simulink model "Bicycle_Rebuild"  (R2019b)
settings: Solver=VariableStepAuto  StartTime=0.0  StopTime=20  MaxStep=1e-3  RelTol=1e-3
values from neighbouring files (symbols this model uses):
  K = lqr(A,B,Q,R)    [Lqr.m]
undefined symbols (not defined in the file or in its folder): DC_Motor, Dynamics, Theta
settings Model: Creator=user  LastModifiedBy=user

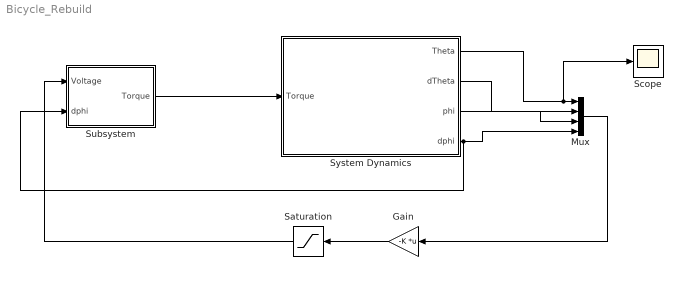
== system Bicycle_Rebuild ==
  Gain : Gain  Gain=-K  Multiplication=Matrix(K*u)
  Mux : Mux
  Saturation : Saturate  UpperLimit=24  LowerLimit=-24
  Scope : Scope
  Subsystem : Subsystem
  System Dynamics : Subsystem
  wires:
  Subsystem/1(Torque) -> System Dynamics/1(Torque)
  System Dynamics/4(dphi) -> Subsystem/2(dphi), Mux/4
  Mux/1 -> Gain/1
  System Dynamics/3(phi) -> Mux/3
  System Dynamics/2(dTheta) -> Mux/2
  System Dynamics/1(Theta) -> Scope/1, Mux/1
  Gain/1 -> Saturation/1
  Saturation/1 -> Subsystem/1(Voltage)

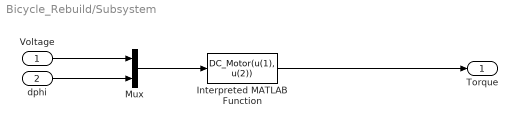
== system Bicycle_Rebuild/Subsystem ==
  Voltage : Inport
  dphi : Inport  Port=2
  Interpreted MATLAB Function : MATLABFcn  MATLABFcn=DC_Motor(u(1), u(2))
  Mux : Mux  Inputs=2
  Torque : Outport
  wires:
  dphi/1 -> Mux/2
  Interpreted MATLAB Function/1 -> Torque/1
  Mux/1 -> Interpreted MATLAB Function/1
  Voltage/1 -> Mux/1

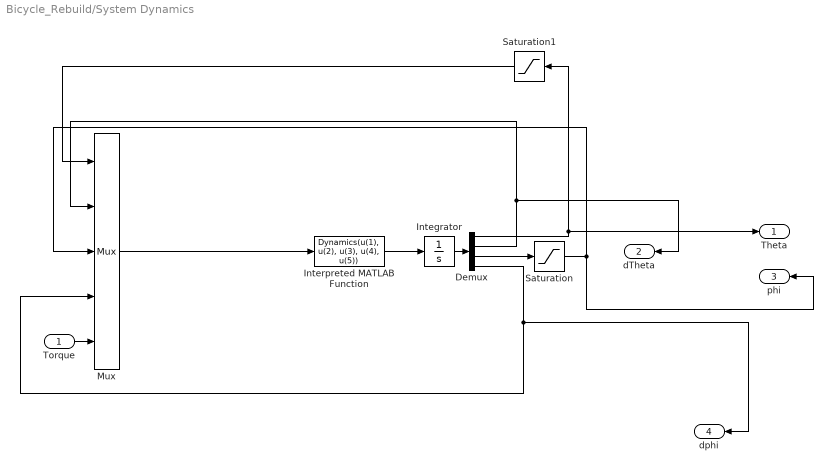
== system Bicycle_Rebuild/System Dynamics ==
  Torque : Inport
  Demux : Demux
  Integrator : Integrator  InitialCondition=[Theta 0 0 0]
  Interpreted MATLAB Function : MATLABFcn  MATLABFcn=Dynamics(u(1), u(2), u(3), u(4), u(5))  OutputDimensions=4
  Mux : Mux  Inputs=5
  Saturation : Saturate  UpperLimit=pi/2  LowerLimit=-pi/2
  Saturation1 : Saturate  UpperLimit=pi/2  LowerLimit=-pi/2
  Theta : Outport
  dTheta : Outport  Port=2
  phi : Outport  Port=3
  dphi : Outport  Port=4
  wires:
  Demux/1 -> Theta/1, Saturation1/1
  Demux/2 -> dTheta/1, Mux/2
  Mux/1 -> Interpreted MATLAB Function/1
  Torque/1 -> Mux/5
  Interpreted MATLAB Function/1 -> Integrator/1
  Integrator/1 -> Demux/1
  Demux/3 -> Saturation/1
  Demux/4 -> Mux/4, dphi/1
  Saturation/1 -> phi/1, Mux/3
  Saturation1/1 -> Mux/1
